simulink model "constellation"  (Simulink 6.6)
settings: Solver=VariableStepDiscrete  StartTime=0.0  StopTime=512/28e6  RelTol=1e-3
StopFcn:
  | figure(2)
  | hold off
  | plot(I_channel,Q_channel,'ko','MarkerFaceColor','b');
  | hold on
  | plot(I_channel_q,Q_channel_q,'ko','MarkerFaceColor','r');
  | legend('Original','Quantised',4);
  | xlabel('I channel');
  | ylabel('Q_channel');
  | title('64 QAM Constellation');
settings Model: Creator=lcrockett  LastModifiedBy=lcrockett
settings OptimizationCC: InlineParams=on  InlineInvariantSignals=on
settings DebuggingCC: SignalResolutionControl=TryResolveAllWithWarning  MultiTaskDSMMsg=warning  MultiTaskCondExecSysMsg=none  StrictBusMsg=None
settings RTWCC: IncludeERTFirstTime=on

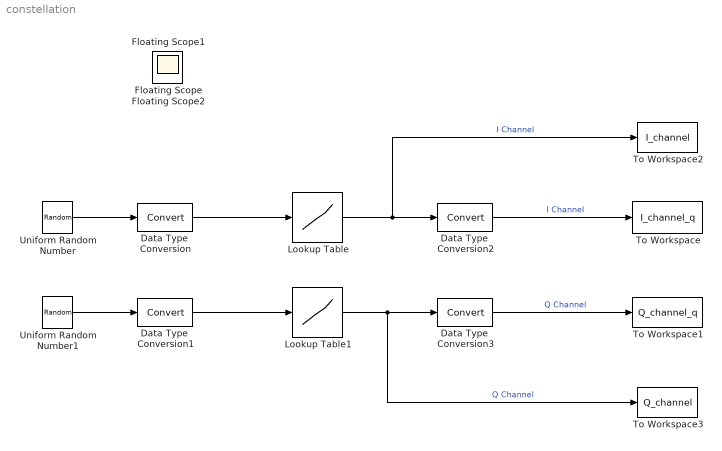
== system constellation ==
  Data Type  Conversion : DataTypeConversion  OutDataTypeMode=Specify via dialog  OutDataType=uint(3)  RndMeth=Nearest  SaturateOnIntegerOverflow=on
  Data Type  Conversion1 : DataTypeConversion  OutDataTypeMode=Specify via dialog  OutDataType=uint(3)  RndMeth=Nearest  SaturateOnIntegerOverflow=on
  Data Type  Conversion2 : DataTypeConversion  OutDataTypeMode=Specify via dialog  OutDataType=sfix(8)  SaturateOnIntegerOverflow=on  RndMeth=Zero
  Data Type  Conversion3 : DataTypeConversion  OutDataTypeMode=Specify via dialog  OutDataType=sfix(8)  SaturateOnIntegerOverflow=on  RndMeth=Zero
  Lookup Table : Lookup  InputValues=[0 1 2 3 4 5 6 7]  OutputValues=[127 90.71428571 54.42857143 18.14285714 -18.14285714 -54.42857143 -90.71428571 -127]  OutDataTypeMode=Specify via dialog  OutDataType=float('double')
  Lookup Table1 : Lookup  InputValues=[0 1 2 3 4 5 6 7]  OutputValues=[127 90.71428571 54.42857143 18.14285714 -18.14285714 -54.42857143 -90.71428571 -127]  OutDataTypeMode=Specify via dialog  OutDataType=float('double')
  To Workspace : ToWorkspace  VariableName=I_channel_q  SampleTime=-1  SaveFormat=Array
  To Workspace1 : ToWorkspace  VariableName=Q_channel_q  SampleTime=-1  SaveFormat=Array
  To Workspace2 : ToWorkspace  VariableName=I_channel  SampleTime=-1  SaveFormat=Array
  To Workspace3 : ToWorkspace  VariableName=Q_channel  SampleTime=-1  SaveFormat=Array
  Uniform Random Number : UniformRandomNumber  Minimum=0  Maximum=7  SampleTime=1/28e6
  Uniform Random Number1 : UniformRandomNumber  Minimum=0  Maximum=7  Seed=1  SampleTime=1/28e6
  Floating Scope : Scope
      settings: Floating=on  YMin=-150  YMax=150
  Floating Scope1 : Scope
      settings: Floating=on
  Floating Scope2 : Scope
      settings: Floating=on
  wires:
  Uniform Random Number/1 -> Data Type  Conversion/1
  Data Type  Conversion1/1 -> Lookup Table1/1
  Uniform Random Number1/1 -> Data Type  Conversion1/1
  Data Type  Conversion/1 -> Lookup Table/1
  Lookup Table/1 -> Data Type  Conversion2/1, To Workspace2/1  "I Channel"
  Lookup Table1/1 -> Data Type  Conversion3/1, To Workspace3/1  "Q Channel"
  Data Type  Conversion2/1 -> To Workspace/1  "I Channel"
  Data Type  Conversion3/1 -> To Workspace1/1  "Q Channel"
